simulink model "regcontrol_model"  (R2016b)
settings: Solver=VariableStepAuto  StartTime=0.0  StopTime=10.0  RelTol=1e-3
settings Model: Creator=Michael Girbino  LastModifiedBy=Michael Girbino

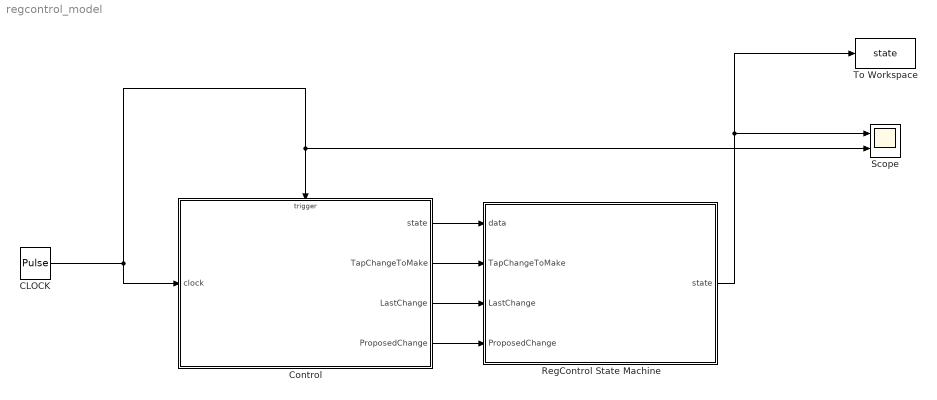
== system regcontrol_model ==
  CLOCK : DiscretePulseGenerator  PulseType=Time based  Period=1  PulseWidth=5
  Control : Stateflow chart  TreatAsAtomicUnit=on
  RegControl State Machine : Stateflow chart  TreatAsAtomicUnit=on
  Scope : Scope  NumInputPorts=2
  To Workspace : ToWorkspace  VariableName=state  SaveFormat=Timeseries  SampleTime=-1
  wires:
  CLOCK/1 -> Control/Trigger, Scope/2, Control/1(clock)
  RegControl State Machine/1(state) -> To Workspace/1, Scope/1
  Control/1(state) -> RegControl State Machine/1(data)
  Control/2(TapChangeToMake) -> RegControl State Machine/2(TapChangeToMake)
  Control/3(LastChange) -> RegControl State Machine/3(LastChange)
  Control/4(ProposedChange) -> RegControl State Machine/4(ProposedChange)

== stateflow chart regcontrol_model/Control ==
  settings: executeAtInitialization=1
  state DoPendingAction
    entry:GetChangeMode(ControlMode);
    state AtLeastOneTap
      entry:
      NumTaps = floor(0.7*ProposedChange/Increment);
      state SteadyState
      state OneTap
        entry:
        NumTaps = 1;
      state SetLastChange
        entry:
        LastChange = NumTaps;
      state NegativeIncrement
        entry:
        TapChangeToMake = -1*NumTaps*Increment;
        LastChange = -1*NumTaps;
      state PositiveIncrement
        entry:
        TapChangeToMake = NumTaps*Increment;
      (default) -> DoPendingAction.AtLeastOneTap.SteadyState
      DoPendingAction.AtLeastOneTap.SteadyState -> OneTap [order 1] : [NumTaps == 0]
      DoPendingAction.AtLeastOneTap.SteadyState -> SetLastChange [order 2] : [NumTaps ~= 0]
      OneTap -> SetLastChange : [NumTaps == 1]
      SetLastChange -> PositiveIncrement [order 1] : [ProposedChange > 0.0]
      SetLastChange -> NegativeIncrement [order 2] : [ProposedChange <= 0.0]
    state OneInDirectionOf
      entry: LastChange = 0;
      state SteadyState
      state ProposeIncrease
        entry:
        MakeChange(ProposedChange, Increment, 1);
      state ProposeDecrease
        during:
        MakeChange(ProposedChange, Increment, -1);
      state ProposeNoChange
        entry: ProposedChange = 0.0;
      (default) -> DoPendingAction.OneInDirectionOf.SteadyState
      DoPendingAction.OneInDirectionOf.SteadyState -> ProposeIncrease [order 1] : [ProposedChange > 0.0]
      (junction 46) -> DoPendingAction.OneInDirectionOf.SteadyState : [abs(ProposedChange) >= 0.9*Increment]
      DoPendingAction.OneInDirectionOf.SteadyState -> ProposeDecrease [order 2] : [ProposedChange <= 0.0]
      ProposeIncrease -> (junction 46) [order 1]
      ProposeDecrease -> (junction 46) [order 2]
      ProposeIncrease -> (junction 42) [order 2]
      ProposeDecrease -> (junction 42) [order 1]
      (junction 42) -> ProposeNoChange : [abs(ProposedChange) < 0.9*Increment]
    (default) -> OneInDirectionOf
    OneInDirectionOf -> AtLeastOneTap : [Change == ChangeModes.Single]
    AtLeastOneTap -> OneInDirectionOf : [Change == ChangeModes.Multiple]
  state GetChangeMode(ControlMode) [function]
    (default) -> (junction 72) : % ControlMode determines single or multiple tap changes
    (junction 72) -> (junction 73) [order 1] : [ControlMode == ControlModes.Static]
    (junction 72) -> (junction 74) [order 2] : {Change = ChangeModes.Multiple;}
    (junction 73) -> (junction 75) : {Change = ChangeModes.Single;}
    (junction 75) -> (junction 74)
    (junction 74) -> (junction 76)
  state MakeChange(ProposedChange, Increment, Direction) [function]
    (default) -> (junction 78)
    (junction 78) -> (junction 86) : {TapChangeToMake = Direction*Increment;
        | LastChange = Direction;
        | ProposedChange = ProposedChange + TapChangeToMake;}
  state Sleep
  Sleep -> DoPendingAction : CLOCK
  DoPendingAction -> Sleep : CLOCK
  (default) -> Sleep
  data: ControlMode function_input; ProposedChange function_input; Increment function_input; Direction function_input; clock input; state output; TapChangeToMake output; LastChange output; ProposedChange output
  events: CLOCK input RISING_EDGE_EVENT

== stateflow chart regcontrol_model/RegControl State Machine ==
  settings: executeAtInitialization=1
  state DeterminePowerForwardDirection
    (junction 144) -> (junction 132) [order 1] : [~ReversePending]
    (junction 144) -> (junction 139) [order 2]
    (junction 132) -> (junction 130) : {action1}
    (junction 130) -> (junction 138) [order 1] : [FwdPower > RevPowerThreshold]
    (junction 130) -> (junction 137) [order 2]
    (junction 138) -> (junction 136) : {ReversePending = true;}
    (junction 137) -> (junction 139)
    (junction 136) -> (junction 137)
    (junction 139) -> (junction 147)
    (junction 147) -> (junction 154) [order 1] : [ReversePending && FwdPower <= RevPowerThreshold]
    (junction 147) -> (junction 151) [order 2] : {action2}
    (junction 154) -> (junction 148) : {% Reset ReversePending;}
    (junction 148) -> (junction 151)
  state DetermineReversal
    (junction 106) -> (junction 107) [order 1] : [~ReversePending]
    (junction 106) -> (junction 110) [order 2]
    (junction 107) -> (junction 108) : {action1}
    (junction 108) -> (junction 109) [order 1] : [FwdPower < (-1*RevPowerThreshold)]
    (junction 108) -> (junction 111) [order 2]
    (junction 109) -> (junction 112) : {ReversePending = true;}
    (junction 111) -> (junction 110)
    (junction 112) -> (junction 111)
    (junction 110) -> (junction 120)
    (junction 120) -> (junction 121) [order 1] : [ReversePending && FwdPower >= (-1*RevPowerThreshold)]
    (junction 120) -> (junction 122) [order 2] : {action2}
    (junction 121) -> (junction 123) : {% Reset ReversePending;}
    (junction 123) -> (junction 122)
  state ReverseNeutralCase
    (junction 175) -> (junction 184) [order 1] : [ReverseNeutral]
    (junction 175) -> (junction 174) [order 2]
    (junction 184) -> (junction 166)
    (junction 166) -> (junction 155) [order 1] : [~Armed]
    (junction 166) -> (junction 165) [order 2]
    (junction 155) -> (junction 160) : {PendingTapChange = 0.0;}
    (junction 160) -> (junction 167) [order 1] : [abs(PresentTap[TapWinding] - 1.0) < EPSILON]
    (junction 160) -> (junction 170) [order 2]
    (junction 167) -> (junction 164) : {Increment = TapIncrement(TapWinding);}
    (junction 165) -> (junction 174)
    (junction 170) -> (junction 165)
    (junction 164) -> (junction 170)
  (default) -> (junction 207) : {ControlledTransformer = TTransfObj(ControlledElement);}
  (junction 207) -> (junction 208) [order 2] : [TapLimitPerChange == 0]
  (junction 208) -> (junction 86) : {PendingTapChange = 0;}
  (junction 207) -> (junction 212) [order 1]
  (junction 86) -> (junction 87) [order 1] : [~UsingRegulatedBus]
  (junction 87) -> (junction 61)
  (junction 86) -> (junction 88) [order 2]
  (junction 61) -> (junction 62) [order 1] : [IsReversible || CogenEnabled]
  (junction 61) -> (junction 65) [order 2]
  (junction 62) -> (junction 63) : {action1}
  (junction 63) -> (junction 64) [order 1] : [If LookingForward && ~InCogenMode]
  (junction 63) -> (junction 144) [order 2] : % If reversed, check if power is back in forward direction
  (junction 64) -> (junction 106) : % Should we reverse?
  (junction 151) -> (junction 175)
  (junction 65) -> (junction 88)
  (junction 127) -> (junction 65)
  (junction 67) -> (junction 127)
  (junction 88) -> (junction 75)
  (junction 122) -> (junction 67)
  (junction 174) -> (junction 127)
  (junction 75) -> (junction 76) [order 1] : [UsingRegulatedBus]
  (junction 75) -> (junction 77) [order 2] : {TransformerConnection = ControlledTransformer.Winding;}
  (junction 76) -> (junction 78) : {}
  (junction 78) -> (junction 77)
  (junction 77) -> (junction 79)
  (junction 212) -> (junction 79)
  data: data input; state output; TapChangeToMake input; LastChange input; ProposedChange input
